simulink model "FullWaveRectifierCT"  (R2024a)
settings: Solver=VariableStepAuto  StartTime=0.0  StopTime=0.1  RelTol=1e-3
libraries: fl_lib x9, nesl_utility x3, ee_lib x1
settings Model: Creator=callie  LastModifiedBy=callie
settings DataIOCC: SignalLogging=off  ReturnWorkspaceOutputs=off  SignalLoggingName=FWRectData
settings SimscapeCC: SimscapeLogType=all  SimscapeLogLimitData=off

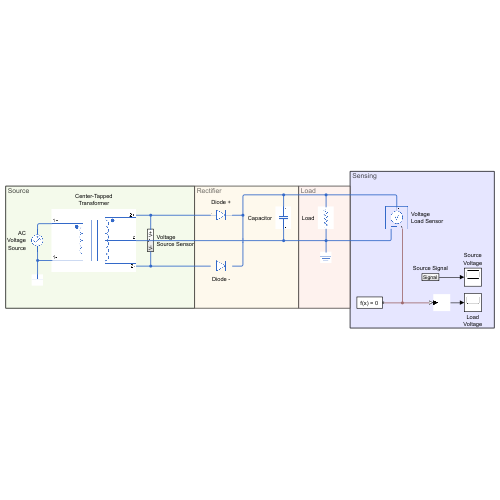
[thumbnail: Simulink's stored preview of the top-level diagram]
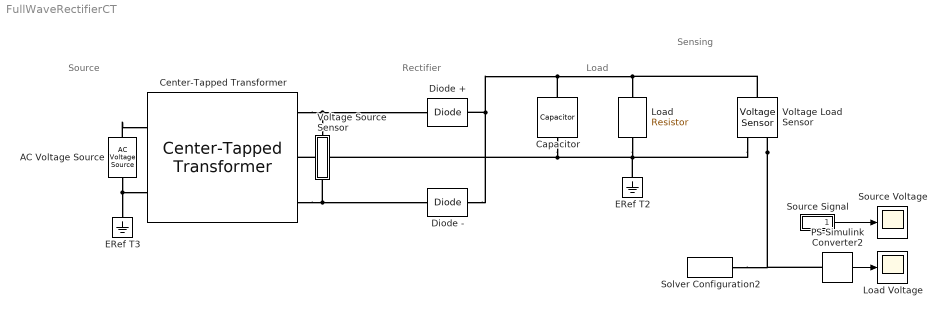
== system FullWaveRectifierCT ==
  note: Source
  note: Rectifier
  note: Load
  note: Sensing
  AC Voltage Source : fl_lib/Electrical/Electrical Sources/AC Voltage Source  amp=sqrt(2)*120 V  shift=0 deg  frequency=60 Hz
  Capacitor : fl_lib/Electrical/Electrical Elements/Capacitor  c=1e-6 F  r=1e-6 Ohm  g=0 1/Ohm  i_specify=off  i_priority=None  i=0 A  i_nominal_specify=off  i_nominal_value=1  i_nominal_unit=A  v_specify=off  v_priority=None  v=0 V  v_nominal_specify=off  v_nominal_value=1  v_nominal_unit=V  vc_specify=off  vc_priority=High  vc=0 V  vc_nominal_specify=off  vc_nominal_value=1  vc_nominal_unit=V
  Center-Tapped Transformer : ee_lib/Passive/Transformers/Center-Tapped Transformer  modeling_option=ee.enum.transformer_option.ideal  n=14  T=0.5  Rw1=0.01 Ohm  L1=0.0001 H  Rw2=0.01 Ohm  L2=0.0001 H  Rm=100 Ohm  Lm=0.04 H  i1_specify=off  i1_priority=None  i1=0 A  i1_nominal_specify=off  i1_nominal_value=1  i1_nominal_unit=A  i2p_specify=off  i2p_priority=None  i2p=0 A  i2p_nominal_specify=off  i2p_nominal_value=1  i2p_nominal_unit=A  i2n_specify=off  i2n_priority=None  i2n=0 A  i2n_nominal_specify=off  i2n_nominal_value=1  i2n_nominal_unit=A
      settings: InternalSimscapePortConfiguration="{\"Bottom\":[],\"Left\":[{\"id\":\"p1\",\"label\":\"1+\",\"type\":\"foundation.electrical.electrical\"},{\"id\":\"n1\",\"label\":\"1-\",\"type\":\"foundation.electrical.electrical\"}],\"Right\":[{\"id\":\"p2\",\"label\":\"2+\",\"type\":\"foundation.electrical.electrical\"},{\"id\":\"c\",\"label\":\"c\",\"type\":\"foundation.electrical.electrical\"},{\"id\":\"n2\",\"label\":\"2-\",\"type\":\"foundation.electrical.electrical\"}],\"Top\":[]}"
  Diode + : fl_lib/Electrical/Electrical Elements/Diode  Vf=0.6 V  Ron=0.3 Ohm  Goff=1e-08 1/Ohm  i_specify=off  i_priority=High  i=0 A  i_nominal_specify=off  i_nominal_value=1  i_nominal_unit=A  v_specify=off  v_priority=High  v=0 V  v_nominal_specify=off  v_nominal_value=1  v_nominal_unit=V
  Diode - : fl_lib/Electrical/Electrical Elements/Diode  Vf=0.6 V  Ron=0.3 Ohm  Goff=1e-08 1/Ohm  i_specify=off  i_priority=High  i=0 A  i_nominal_specify=off  i_nominal_value=1  i_nominal_unit=A  v_specify=off  v_priority=High  v=0 V  v_nominal_specify=off  v_nominal_value=1  v_nominal_unit=V
  ERef T2 : fl_lib/Electrical/Electrical Elements/Electrical Reference
  ERef T3 : fl_lib/Electrical/Electrical Elements/Electrical Reference
  Load : fl_lib/Electrical/Electrical Elements/Resistor  R=100 Ohm  i_specify=off  i_priority=High  i=0 A  i_nominal_specify=off  i_nominal_value=1  i_nominal_unit=A  v_specify=off  v_priority=High  v=0 V  v_nominal_specify=off  v_nominal_value=1  v_nominal_unit=V
  Load Voltage : Scope
  PS-Simulink Converter2 : nesl_utility/PS-Simulink Converter  PhysicalDomain=network_engine_domain  SubClassName=ps_output  LeftPortType=input  RightPortType=output  PseudoPeriodic=off  Frequencies=[]  VectorFormat=1-D array  Unit=inherit  AffineConversion=off
  Solver Configuration2 : nesl_utility/Solver Configuration  PhysicalDomain=network_engine_domain  SubClassName=solver  LeftPortType=input  RightPortType=generic  Tones=[]  Harmonics=[]  SimulateNoise=off  Profile=off  UseLocalSampling=off  EnableSwitchedLinearOptims=on  FrequencyDomain=off  UseCCode=off  RelTol=0.001  AbsTol=1e-06  MinStep=1e-09  ToWorkspace=off  RevertToSquareIcSolve=off  NumHomotopyIterations=100  PhasorMode=off  PhasorModeNumHarmonics=1  ConsistencySolver=NEWTON_XTOL_AFTER_FTOL  IndexReductionMethod=DerivativeReplacement  DoDC=off  ResidualTolerance=1e-9  ConsistencyTolSource=GLOBAL  ConsistencyAbsTol=0.001  ConsistencyRelTol=0.001  ConsistencyTolFactor=0.001  UseLocalSolver=off  LocalSolverChoice=NE_BACKWARD_EULER_ADVANCER  ResolveIndetEquations=on  FunctionEvalNumThread=1  LocalSolverSampleTime=.001  DoFixedCost=off  MaxNonlinIter=3  MaxModeIter=2  ComputeImpulses=off  ImpulseIterations=2  LinearAlgebra=auto  LinearAlgebraNumThread=0  EquationFormulation=NE_TIME_EF  DelaysMemoryBudget=1024  AutomaticFiltering=on  FilteringTimeConstant=0.001  PartitionStorageMethod=AS_NEEDED  PartitionMemoryBudget=1024  PartitionMethod=FAST  MultibodyUseLocalSolver=off  MultibodyLocalSolverChoice=ODE1  MultibodyLocalSolverSampleTime=0.001
  Source Voltage : Scope
  Source Signal : Subsystem
  Voltage Load Sensor : fl_lib/Electrical/Electrical Sensors/Voltage Sensor
  Voltage Source Sensor : Subsystem
  wires:
  PS-Simulink Converter2/1 -> Load Voltage/1
  Source Signal/1(Signal) -> Source Voltage/1
  connections:
  AC Voltage Source/RConn1 -- Center-Tapped Transformer/LConn2 -- ERef T3/LConn1
  AC Voltage Source/LConn1 -- Center-Tapped Transformer/LConn1
  Center-Tapped Transformer/RConn1 -- Diode +/LConn1 -- Voltage Source Sensor/LConn1
  Center-Tapped Transformer/RConn3 -- Diode -/LConn1 -- Voltage Source Sensor/RConn1
  Voltage Load Sensor/RConn1 -- Solver Configuration2/RConn1 -- PS-Simulink Converter2/LConn1
  Diode -/RConn1 -- Voltage Load Sensor/LConn1 -- Load/LConn1 -- Capacitor/LConn1 -- Diode +/RConn1
  Load/RConn1 -- Voltage Load Sensor/RConn2 -- ERef T2/LConn1 -- Capacitor/RConn1 -- Center-Tapped Transformer/RConn2

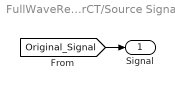
== system FullWaveRectifierCT/Source Signal ==
  Signal : Outport
  wires:
  [Original_Signal] -> Signal/1

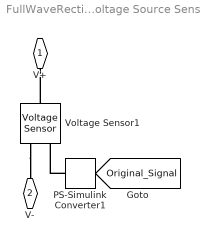
== system FullWaveRectifierCT/Voltage Source Sensor ==
  PS-Simulink Converter1 : nesl_utility/PS-Simulink Converter  PhysicalDomain=network_engine_domain  SubClassName=ps_output  LeftPortType=input  RightPortType=output  PseudoPeriodic=off  Frequencies=[]  VectorFormat=1-D array  Unit=inherit  AffineConversion=off
  Voltage Sensor1 : fl_lib/Electrical/Electrical Sensors/Voltage Sensor
  V+ : PMIOPort  Side=Left
  V- : PMIOPort  Port=2  Side=Right
  tag scope: Original_Signal=global
  wires:
  PS-Simulink Converter1/1 -> [Original_Signal]
  connections:
  PS-Simulink Converter1/LConn1 -- Voltage Sensor1/RConn1
  Voltage Sensor1/LConn1 -- V+/RConn1
  Voltage Sensor1/RConn2 -- V-/RConn1
